simulink library "common_lib"  (R2018b)
settings: Solver=VariableStepAuto  StartTime=0.0  StopTime=10.0  RelTol=1e-3
libraries: $bdroot x1
settings Model: Creator=F074018  LastModifiedBy=F074018

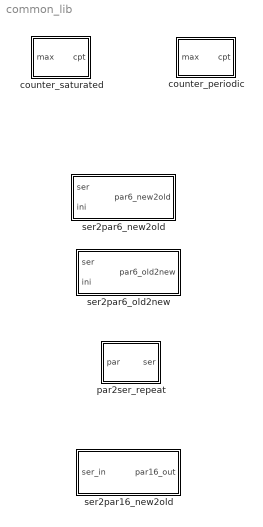
== system common_lib ==
  counter_periodic : Subsystem
  counter_saturated : Subsystem
  par2ser_repeat : Subsystem
  ser2par16_new2old : Subsystem
  ser2par6_new2old : Subsystem
  ser2par6_old2new : Subsystem

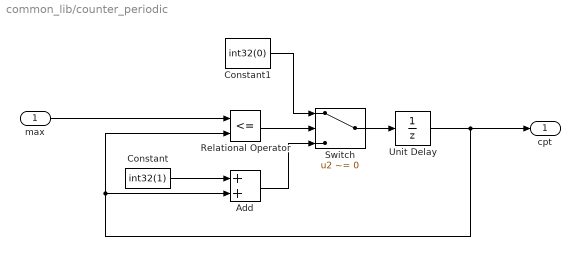
== system common_lib/counter_periodic ==
  max : Inport
  Add : Sum  InputSameDT=on  OutDataTypeStr=Inherit: Same as first input
  Constant : Constant  Value=int32(1)
  Constant1 : Constant  Value=int32(0)
  Relational Operator : RelationalOperator  Operator=<=  OutDataTypeStr=boolean  RndMeth=Simplest
  Switch : Switch  Criteria=u2 ~= 0  InputSameDT=on
  Unit Delay : UnitDelay  InitialCondition=int32(0)  SampleTime=-1
      settings: AttributesFormatString=%<InitialCondition>
  cpt : Outport
  wires:
  Unit Delay/1 -> Add/2, Relational Operator/2, cpt/1
  Constant/1 -> Add/1
  Add/1 -> Switch/3
  Switch/1 -> Unit Delay/1
  Relational Operator/1 -> Switch/2
  Constant1/1 -> Switch/1
  max/1 -> Relational Operator/1

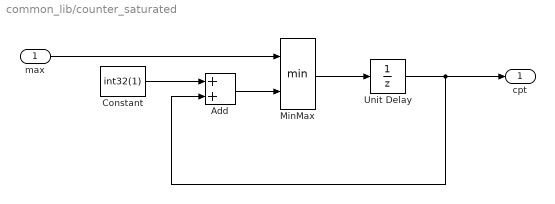
== system common_lib/counter_saturated ==
  max : Inport
  Add : Sum  InputSameDT=on  OutDataTypeStr=Inherit: Same as first input
  Constant : Constant  Value=int32(1)
  MinMax : MinMax  Inputs=2
  Unit Delay : UnitDelay  InitialCondition=int32(0)  SampleTime=-1
      settings: AttributesFormatString=%<InitialCondition>
  cpt : Outport
  wires:
  Unit Delay/1 -> Add/2, cpt/1
  Constant/1 -> Add/1
  Add/1 -> MinMax/2
  max/1 -> MinMax/1
  MinMax/1 -> Unit Delay/1

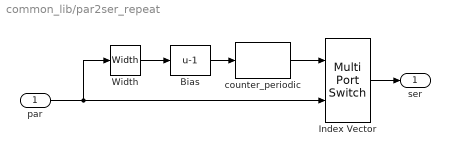
== system common_lib/par2ser_repeat ==
  par : Inport
  Bias : Bias  Bias=-1
  Index Vector : MultiPortSwitch  DataPortOrder=Zero-based contiguous  Inputs=1  zeroidx=on
  Width : Width
  counter_periodic : $bdroot/counter_periodic  SystemSampleTime=-1
  ser : Outport
  wires:
  par/1 -> Index Vector/2, Width/1
  counter_periodic/1 -> Index Vector/1
  Index Vector/1 -> ser/1
  Bias/1 -> counter_periodic/1
  Width/1 -> Bias/1

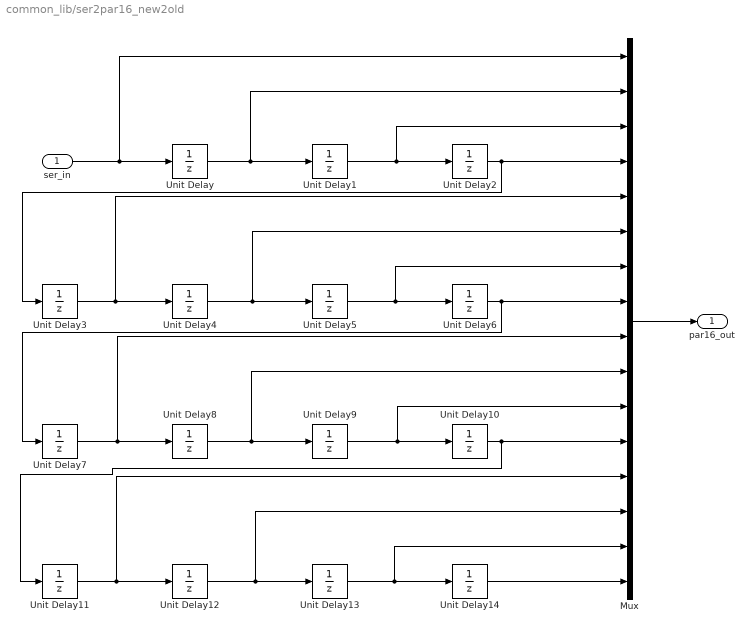
== system common_lib/ser2par16_new2old ==
  ser_in : Inport
  Mux : Mux  Inputs=16
  Unit Delay{,1..14} (15 alike) : UnitDelay  SampleTime=-1
      settings: AttributesFormatString=%<InitialCondition>
  par16_out : Outport
  wires:
  ser_in/1 -> Mux/1, Unit Delay/1
  Unit Delay/1 -> Mux/2, Unit Delay1/1
  Unit Delay1/1 -> Mux/3, Unit Delay2/1
  Unit Delay5/1 -> Mux/7, Unit Delay6/1
  Unit Delay4/1 -> Mux/6, Unit Delay5/1
  Unit Delay3/1 -> Mux/5, Unit Delay4/1
  Unit Delay7/1 -> Mux/9, Unit Delay8/1
  Unit Delay9/1 -> Mux/11, Unit Delay10/1
  Unit Delay8/1 -> Mux/10, Unit Delay9/1
  Unit Delay11/1 -> Mux/13, Unit Delay12/1
  Unit Delay13/1 -> Mux/15, Unit Delay14/1
  Unit Delay12/1 -> Mux/14, Unit Delay13/1
  Unit Delay2/1 -> Mux/4, Unit Delay3/1
  Unit Delay6/1 -> Unit Delay7/1, Mux/8
  Unit Delay10/1 -> Unit Delay11/1, Mux/12
  Mux/1 -> par16_out/1
  Unit Delay14/1 -> Mux/16

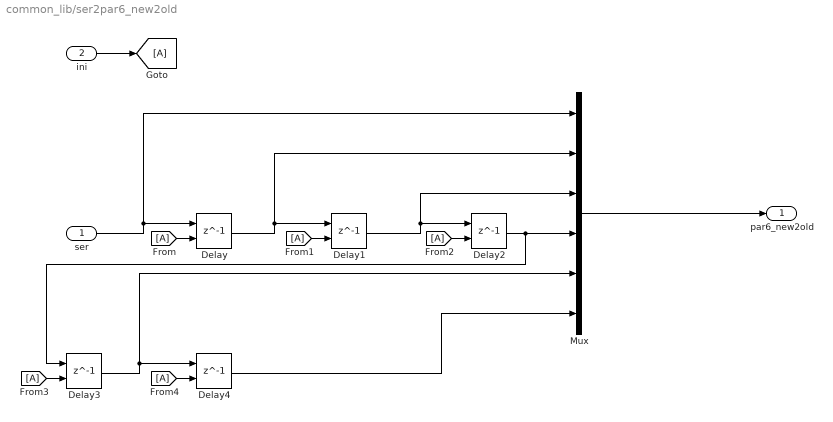
== system common_lib/ser2par6_new2old ==
  ser : Inport
  ini : Inport  Port=2
  Delay{,1..4} (5 alike) : Delay  DelayLength=1  InitialConditionSource=Input port
      settings: InputPortMap=u0,p4
  Mux : Mux  Inputs=6
  par6_new2old : Outport  PortDimensions=6
  wires:
  ser/1 -> Delay/1, Mux/1
  Delay/1 -> Delay1/1, Mux/2
  Delay1/1 -> Delay2/1, Mux/3
  Delay3/1 -> Delay4/1, Mux/5
  Delay2/1 -> Delay3/1, Mux/4
  Delay4/1 -> Mux/6
  Mux/1 -> par6_new2old/1
  ini/1 -> [A]
  [A] -> Delay/2
  [A] -> Delay1/2
  [A] -> Delay2/2
  [A] -> Delay4/2
  [A] -> Delay3/2

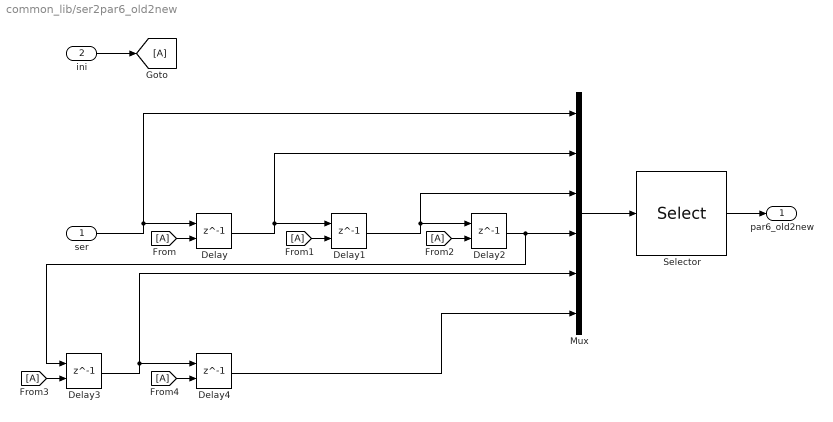
== system common_lib/ser2par6_old2new ==
  ser : Inport
  ini : Inport  Port=2
  Delay{,1..4} (5 alike) : Delay  DelayLength=1  InitialConditionSource=Input port
      settings: InputPortMap=u0,p4
  Mux : Mux  Inputs=6
  Selector : Selector  InputPortWidth=6  IndexOptions=Index vector (dialog)  Indices=6:-1:1  OutputSizes=1
  par6_old2new : Outport  PortDimensions=6
  wires:
  ser/1 -> Delay/1, Mux/1
  Delay/1 -> Delay1/1, Mux/2
  Delay1/1 -> Delay2/1, Mux/3
  Delay3/1 -> Delay4/1, Mux/5
  Delay2/1 -> Delay3/1, Mux/4
  Mux/1 -> Selector/1
  Delay4/1 -> Mux/6
  Selector/1 -> par6_old2new/1
  ini/1 -> [A]
  [A] -> Delay/2
  [A] -> Delay1/2
  [A] -> Delay2/2
  [A] -> Delay4/2
  [A] -> Delay3/2
